simulink model "ejercicio_2_laborarorio_1"  (R2024b)
settings: Solver=VariableStepAuto  StartTime=0.0  StopTime=0.1  RelTol=1e-3
libraries: spsDiodeLib x6, spsSeriesRLCBranchLib x6, spsGroundLib x6, spsRMSLib x6, spsACVoltageSourceLib x3, spsLinearTransformerLib x3, spsMultimeterLib x3, sps_lib x1
settings Model: Creator=desim  LastModifiedBy=desim

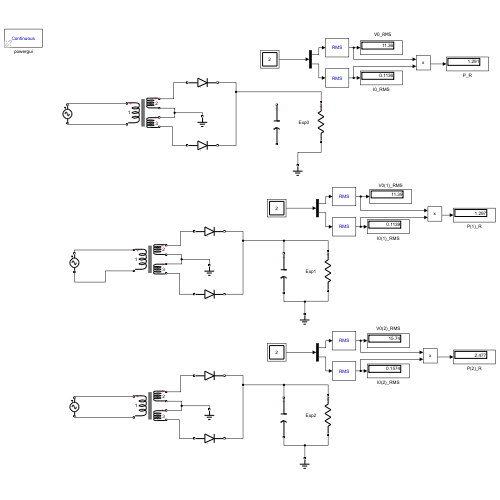
[thumbnail: Simulink's stored preview of the top-level diagram]
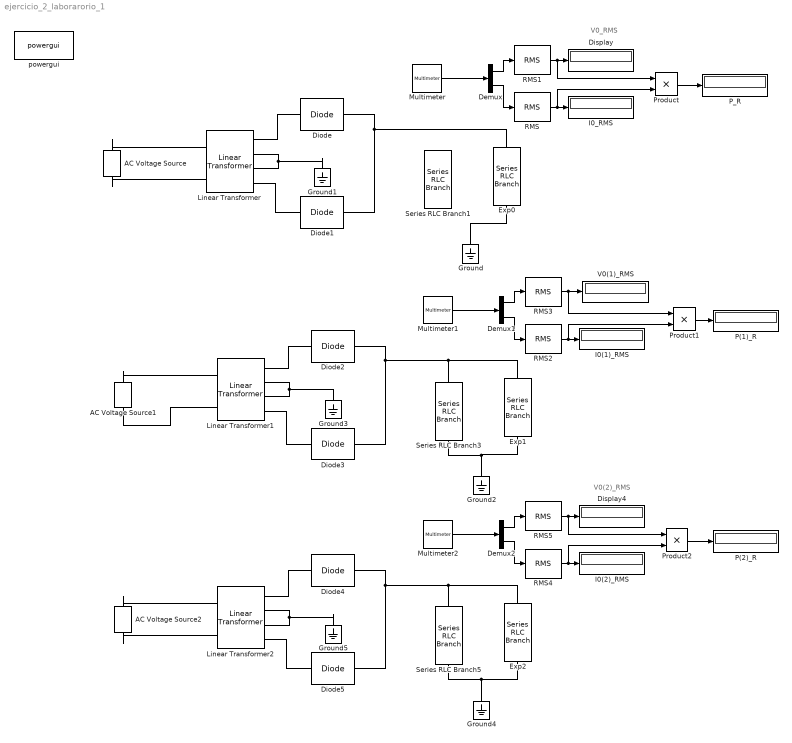
== system ejercicio_2_laborarorio_1 ==
  note: V0(2)_RMS
  note: V0_RMS
  AC Voltage Source : spsACVoltageSourceLib/AC Voltage Source  Amplitude=220*sqrt(2)  Phase=0  Frequency=50  SampleTime=0  Measurements=Voltage  BusType=swing  Pref=10e3  Qref=0  Qmin=-inf  Qmax=+inf
  AC Voltage Source1 : spsACVoltageSourceLib/AC Voltage Source  Amplitude=220*sqrt(2)  Phase=0  Frequency=50  SampleTime=0  Measurements=Voltage  BusType=swing  Pref=10e3  Qref=0  Qmin=-inf  Qmax=+inf
  AC Voltage Source2 : spsACVoltageSourceLib/AC Voltage Source  Amplitude=220*sqrt(2)  Phase=0  Frequency=50  SampleTime=0  Measurements=Voltage  BusType=swing  Pref=10e3  Qref=0  Qmin=-inf  Qmax=+inf
  Demux : Demux  Outputs=2
  Demux1 : Demux  Outputs=2
  Demux2 : Demux  Outputs=2
  Diode{,1..5} (6 alike) : spsDiodeLib/Diode  Ron=0.01  Lon=0  Vf=0.7  IC=0  UseSnubber=0  Rs=inf  Cs=0  Measurements=off
  Display : Display
  Display4 : Display
  Exp0 : spsSeriesRLCBranchLib/Series RLC Branch  LConnTagsString=__new0  RConnTagsString=__new0  BranchType=R  Resistance=100  Inductance=1e-3  SetiL0=off  InitialCurrent=0  Capacitance=1e-6  Setx0=off  InitialVoltage=0  Measurements=Branch voltage and current
  Exp1 : spsSeriesRLCBranchLib/Series RLC Branch  LConnTagsString=__new0  RConnTagsString=__new0  BranchType=R  Resistance=100  Inductance=1e-3  SetiL0=off  InitialCurrent=0  Capacitance=1e-6  Setx0=off  InitialVoltage=0  Measurements=Branch voltage and current
  Exp2 : spsSeriesRLCBranchLib/Series RLC Branch  LConnTagsString=__new0  RConnTagsString=__new0  BranchType=R  Resistance=100  Inductance=1e-3  SetiL0=off  InitialCurrent=0  Capacitance=1e-6  Setx0=off  InitialVoltage=0  Measurements=Branch voltage and current
  Ground{,1..5} (6 alike) : spsGroundLib/Ground  LConnTagsString=a
  I0(1)_RMS : Display
  I0(2)_RMS : Display
  I0_RMS : Display
  Linear Transformer : spsLinearTransformerLib/Linear Transformer  UNITS=SI  NominalPower=[ 12 50 ]  winding1=[220 1 0.01]  winding2=[12 0.1 0.001]  ThreeWindings=on  winding3=[12 0.1 0.001]  RmLm=[1.0804e+06 2866]  Measurements=All voltages and currents  DataType=on
  Linear Transformer1 : spsLinearTransformerLib/Linear Transformer  UNITS=SI  NominalPower=[ 12 50 ]  winding1=[220 1 0.01]  winding2=[12 0.1 0.001]  ThreeWindings=on  winding3=[12 0.1 0.001]  RmLm=[1.0804e+06 2866]  Measurements=All voltages and currents  DataType=on
  Linear Transformer2 : spsLinearTransformerLib/Linear Transformer  UNITS=SI  NominalPower=[ 12 50 ]  winding1=[220 1 0.01]  winding2=[12 0.1 0.001]  ThreeWindings=on  winding3=[12 0.1 0.001]  RmLm=[1.0804e+06 2866]  Measurements=All voltages and currents  DataType=on
  Multimeter : spsMultimeterLib/Multimeter  L=40  sel=[1 18]  yselected={}  Gain=[1 1]  OutputType=Complex  PlotAtSimulationStop=off  PhasorSimulation=off
  Multimeter1 : spsMultimeterLib/Multimeter  L=40  sel=[2 19]  yselected={}  Gain=[1 1]  OutputType=Complex  PlotAtSimulationStop=off  PhasorSimulation=off
  Multimeter2 : spsMultimeterLib/Multimeter  L=40  sel=[3 20]  yselected={}  Gain=[1 1]  OutputType=Complex  PlotAtSimulationStop=off  PhasorSimulation=off
  P(1)_R : Display
  P(2)_R : Display
  P_R : Display
  Product : Product
  Product1 : Product
  Product2 : Product
  RMS{,1..5} (6 alike) : spsRMSLib/RMS  TrueRMS=on  Freq=100  RMSInit=0  Ts=0
  Series RLC Branch1 : spsSeriesRLCBranchLib/Series RLC Branch  LConnTagsString=__new0  RConnTagsString=__new0  BranchType=C  Resistance=1  Inductance=1e-3  SetiL0=off  InitialCurrent=0  Capacitance=0  Setx0=off  InitialVoltage=0  Measurements=Branch voltage and current
  Series RLC Branch3 : spsSeriesRLCBranchLib/Series RLC Branch  LConnTagsString=__new0  RConnTagsString=__new0  BranchType=C  Resistance=1  Inductance=1e-3  SetiL0=off  InitialCurrent=0  Capacitance=10e-6  Setx0=off  InitialVoltage=0  Measurements=Branch voltage and current
  Series RLC Branch5 : spsSeriesRLCBranchLib/Series RLC Branch  LConnTagsString=__new0  RConnTagsString=__new0  BranchType=C  Resistance=1  Inductance=1e-3  SetiL0=off  InitialCurrent=0  Capacitance=1000e-6  Setx0=off  InitialVoltage=0  Measurements=Branch voltage and current
  V0(1)_RMS : Display
  powergui : sps_lib/powergui  Priority=1  SimulationMode=Continuous  SampleTime=50e-6  frequency=60  Iterations=50  frequencyindice=50  Pbase=100e6  ErrMax=1e-4  UnitsV=kV  UnitsW=MW  buscounter=0  FunctionMessages=off  echomessages=off  EnableUseOfTLC=off  CurrentSourceSwitches=off  DisableSnubberDevices=off  DisableRonSwitches=off  DisableVfSwitches=off  DisplayEquations=off  AutomaticDiscreteSolvers=off  SolverType=Tustin/Backward Euler (TBE)  Interpol=off  ExternalGateDelay=off  methode=off  Ts=100  x0status=blocks  SPID=on  SwTol=0  HookPort=off  NonlinearTolerance=1e-4  nMaxIteration=100  ContinueOnMaxIteration=off  RestoreLinks=warning  ResistiveCurrentMeasurement=off  Frange=[0:2:500]  Ylog=off  Xlog=on  ShowGrid=off  save=off  variable=ZData  structure=0  ZoomFFT=off  StartTime=0.0  cycles=1  DisplayStyle=1  fundamental=60  FreqAxis=off  MaxFrequency=1000  frequencyindicesteady=1  RmsSteady=1  display=off
  wires:
  Multimeter/1 -> Demux/1
  RMS/1 -> Product/2, I0_RMS/1
  Demux/2 -> RMS/1
  RMS1/1 -> Product/1, Display/1
  Demux/1 -> RMS1/1
  Demux1/2 -> RMS2/1
  Demux1/1 -> RMS3/1
  RMS2/1 -> Product1/2, I0(1)_RMS/1
  RMS3/1 -> Product1/1, V0(1)_RMS/1
  Multimeter1/1 -> Demux1/1
  Demux2/2 -> RMS4/1
  Demux2/1 -> RMS5/1
  RMS4/1 -> Product2/2, I0(2)_RMS/1
  RMS5/1 -> Product2/1, Display4/1
  Multimeter2/1 -> Demux2/1
  Product/1 -> P_R/1
  Product1/1 -> P(1)_R/1
  Product2/1 -> P(2)_R/1
  connections:
  AC Voltage Source/RConn1 -- Linear Transformer/LConn1
  AC Voltage Source/LConn1 -- Linear Transformer/LConn2
  Diode/LConn1 -- Linear Transformer/RConn1
  Diode1/LConn1 -- Linear Transformer/RConn4
  Ground/LConn1 -- Exp0/RConn1
  Linear Transformer/RConn3 -- Ground1/LConn1 -- Linear Transformer/RConn2
  Diode/RConn1 -- Exp0/LConn1 -- Diode1/RConn1
  Linear Transformer1/RConn3 -- Ground3/LConn1 -- Linear Transformer1/RConn2
  Diode2/RConn1 -- Exp1/LConn1 -- Series RLC Branch3/LConn1 -- Diode3/RConn1
  AC Voltage Source1/LConn1 -- Linear Transformer1/LConn2
  AC Voltage Source1/RConn1 -- Linear Transformer1/LConn1
  Ground2/LConn1 -- Series RLC Branch3/RConn1 -- Exp1/RConn1
  Diode2/LConn1 -- Linear Transformer1/RConn1
  Diode3/LConn1 -- Linear Transformer1/RConn4
  Linear Transformer2/RConn3 -- Ground5/LConn1 -- Linear Transformer2/RConn2
  Diode4/RConn1 -- Series RLC Branch5/LConn1 -- Exp2/LConn1 -- Diode5/RConn1
  AC Voltage Source2/LConn1 -- Linear Transformer2/LConn2
  AC Voltage Source2/RConn1 -- Linear Transformer2/LConn1
  Ground4/LConn1 -- Exp2/RConn1 -- Series RLC Branch5/RConn1
  Diode4/LConn1 -- Linear Transformer2/RConn1
  Diode5/LConn1 -- Linear Transformer2/RConn4
